simulink model "library_test"  (Simulink 7.1)
settings: Solver=FixedStepDiscrete  StartTime=0.0  StopTime=5.0  FixedStep=0.1  RelTol=1e-3
libraries: arduino_io_lib x11, simulink x2
settings Model: Creator=gvallabh  LastModifiedBy=gcampa
settings OptimizationCC: InitFltsAndDblsToZero=off
settings DebuggingCC: StrictBusMsg=ErrorLevel1
settings GRTTargetCC: CPPClassGenCompliant=off

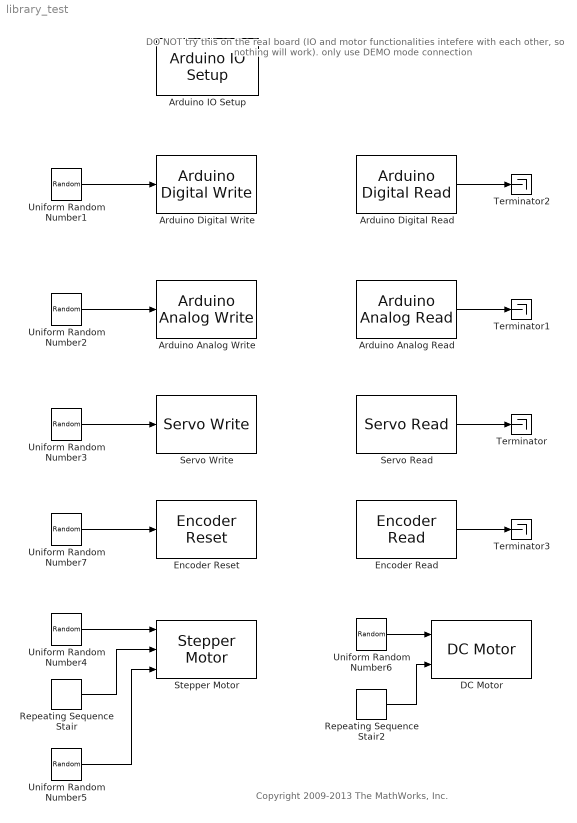
== system library_test ==
  note: DO NOT try this on the real board
      | (IO and motor functionalities intefere
      | with each other, so nothing will work).
      | only use DEMO mode connection
  note: Copyright 2009-2013 The MathWorks, Inc.
  Arduino Analog Read : arduino_io_lib/Arduino Analog Read  arduinoVar=Temporary arduino variable: Arduino1  arduinoPin=0  T=0.1
  Arduino Analog Write : arduino_io_lib/Arduino Analog Write  arduinoVar=Temporary arduino variable: Arduino1  arduinoPin=3  T=-1
  Arduino Digital Read : arduino_io_lib/Arduino Digital Read  arduinoVar=Temporary arduino variable: Arduino1  arduinoPin=2  T=0.1
  Arduino Digital Write : arduino_io_lib/Arduino Digital Write  arduinoVar=Temporary arduino variable: Arduino1  arduinoPin=3  T=-1
  Arduino IO Setup : arduino_io_lib/Arduino IO Setup  Priority=3  arduinoVar=Temporary arduino variable: Arduino1  workspaceVarName=a  comPort=DEMO
  DC Motor : arduino_io_lib/DC Motor  arduinoVar=Temporary arduino variable: Arduino1  motorNum=3  sendOnChange=on  T=-1
  Encoder Read : arduino_io_lib/Encoder Read  arduinoVar=Temporary arduino variable: Arduino1  encNum=1  pinA=3  pinB=2  DbDl=0  T=0.1
  Encoder Reset : arduino_io_lib/Encoder Reset  arduinoVar=Temporary arduino variable: Arduino1  encNum=1  T=0.1
  Repeating Sequence Stair : simulink/Sources/Repeating Sequence Stair  OutValues=[10 10 10 10 20 20 20 20 10].'  tsamp=-1  OutMin=[]  OutMax=[]  OutDataTypeStr=double  OutputDataTypeScalingMode=double  OutDataType=fixdt(0,8)  ConRadixGroup=Best Precision: Vector-wise  OutScaling=2^-12
  Repeating Sequence Stair2 : simulink/Sources/Repeating Sequence Stair  OutValues=[10 10 20 20 20]  tsamp=-1  OutMin=[]  OutMax=[]  OutDataTypeStr=double  OutputDataTypeScalingMode=double  OutDataType=fixdt(0,8)  ConRadixGroup=Best Precision: Vector-wise  OutScaling=2^-12
  Servo Read : arduino_io_lib/Servo Read  arduinoVar=Temporary arduino variable: Arduino1  pinNum=10  T=0.1
  Servo Write : arduino_io_lib/Servo Write  arduinoVar=Temporary arduino variable: Arduino1  pinNum=9  T=-1
  Stepper Motor : arduino_io_lib/Stepper Motor  arduinoVar=Temporary arduino variable: Arduino1  motorNum=1  motionStyle=single  sendOnChange=off  T=-1
  Terminator{,1..3} (4 alike) : Terminator
  Uniform Random Number1 : UniformRandomNumber  Minimum=0  SampleTime=0.1
  Uniform Random Number2 : UniformRandomNumber  Minimum=0  Maximum=255  SampleTime=0.1
  Uniform Random Number3 : UniformRandomNumber  Minimum=0  Maximum=180  SampleTime=0.1
  Uniform Random Number4 : UniformRandomNumber  SampleTime=0.1
  Uniform Random Number5 : UniformRandomNumber  Minimum=0  Maximum=30  SampleTime=0.1
  Uniform Random Number6 : UniformRandomNumber  SampleTime=0.1
  Uniform Random Number7 : UniformRandomNumber  Minimum=0  Maximum=180  SampleTime=0.1
  wires:
  Repeating Sequence Stair/1 -> Stepper Motor/2
  Repeating Sequence Stair2/1 -> DC Motor/2
  Servo Read/1 -> Terminator/1
  Arduino Analog Read/1 -> Terminator1/1
  Arduino Digital Read/1 -> Terminator2/1
  Uniform Random Number3/1 -> Servo Write/1
  Uniform Random Number2/1 -> Arduino Analog Write/1
  Uniform Random Number1/1 -> Arduino Digital Write/1
  Uniform Random Number4/1 -> Stepper Motor/1
  Uniform Random Number5/1 -> Stepper Motor/3
  Uniform Random Number6/1 -> DC Motor/1
  Encoder Read/1 -> Terminator3/1
  Uniform Random Number7/1 -> Encoder Reset/1
